simulink model "app_Main10msMgrrr"  (R2019b)
settings: Solver=FixedStepDiscrete  StartTime=0.0  StopTime=inf  FixedStep=0.01  RelTol=1e-3  EnableMultiTasking=on
PreLoadFcn:
  | try
  |    tapas_types('load');
  | catch
  |   disp('TAPAS WARNING: Tapas Types could not be loaded ...');
  | end
  | 
  | try
  |   app_types('load');
  | catch
  |   currdir =pwd;
  |   try
  |     cd('..\app_types\');
  |     app_types('load');
  |     cd(currdir);
  |   catch
  |     try
  |        cd('..\..\app_types\');
  |        app_types('load');
  |        cd(currdir);
  |     catch
  |        cd(currdir);
  |        disp('TAPAS WARNING: Application Types could not be loaded ...');
  |     end
  |   end
  |   try
  |       clear currdir;
  |   catch
  |      %Do nothing
  |   end
  | end
libraries: Lib_Rev2_Dvcu_IO x44, Lib_Rev2_Dvcu_Anlg x23, simulink x3, hdlsllib x1
settings Model: Creator=kmansour  LastModifiedBy=User
settings DataIOCC: LimitDataPoints=on  SaveFormat=Array  ReturnWorkspaceOutputs=off
settings OptimizationCC: LifeSpan=1  EfficientTunableParamExpr=on
settings DebuggingCC: AllowSymbolicDim=off  SFUnexpectedBacktrackingDiag=warning  SFNoUnconditionalDefaultTransitionDiag=warning  SFExecutionAtInitializationDiag=none  ArithmeticOperatorsInVariantConditions=warning
settings HardwareCC: ProdBitPerPointer=32  ProdBitPerSizeT=32  ProdBitPerPtrDiffT=32  ProdLargestAtomicInteger=Long  ProdLargestAtomicFloat=Double  ProdEndianess=BigEndian  ProdWordSize=32  ProdHWDeviceType=Texas Instruments->TMS570 Cortex-R4
settings ModelReferenceCC: ModelReferenceNumInstancesAllowed=Single  PropagateSignalLabelsOutOfModel=off
settings SFSimCC: SimUseLocalCustomCode=off  MATLABDynamicMemAlloc=off  CustomCodeUndefinedFunction=UseInterfaceOnly
settings RTWCC: SystemTargetFile=ert.tlc  GenCodeOnly=on  TemplateMakefile=ert_default_tmf  GenerateReport=on  RTWUseLocalCustomCode=off  IncludeHyperlinkInReport=on  LaunchReport=on  GenerateTraceInfo=on  GenerateTraceReport=on  GenerateTraceReportSl=on  GenerateTraceReportSf=on  GenerateTraceReportEml=on  CheckMdlBeforeBuild=Warning
settings CodeAppCC: IgnoreCustomStorageClasses=off  MaxIdLength=63  StateflowObjectComments=on
settings ERTTargetCC: MultiwordLength=2048  GenerateSampleERTMain=on  SuppressErrorStatus=on  GenerateASAP2=on  RTWCAPISignals=on  RTWCAPIParams=on  RTWCAPIStates=on  RTWCAPIRootIO=on  ERTSrcFileBannerTemplate=deMCD_code_template.cgt  ERTHdrFileBannerTemplate=deMCD_code_template.cgt  ERTDataSrcFileTemplate=deMCD_code_template.cgt  ERTDataHdrFileTemplate=deMCD_code_template.cgt  ERTCustomFileTemplate=example_file_process.tlc  ConvertIfToSwitch=off  SuppressUnreachableDefaultCases=off
settings ConfigComp: CovMetricSettings=dw  CovHtmlReporting=on  CovSaveCumulativeToWorkspaceVar=on  CovSaveSingleToWorkspaceVar=on  CovExternalEMLEnable=off

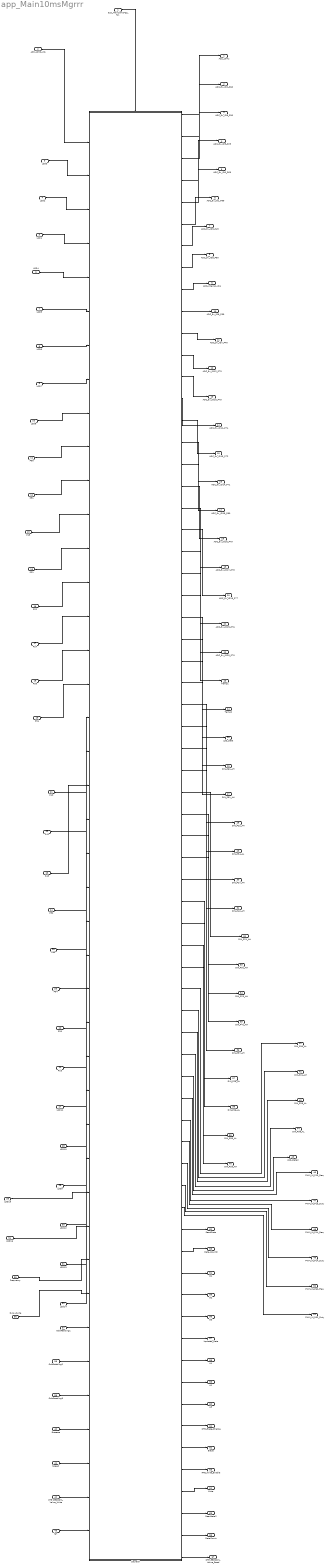
== system app_Main10msMgrrr ==
  app_Main10msMgr_fcn : Inport  SampleTime=10e-3  OutputFunctionCall=on
  APP_10MS_IN1 : Inport  Port=2
  LSD3 : Inport  Port=3
  LSD2 : Inport  Port=4
  LSD1 : Inport  Port=5
  LSD4 : Inport  Port=6
  LSD5 : Inport  Port=7
  LSD6 : Inport  Port=8
  LSD7 : Inport  Port=9
  LSD8 : Inport  Port=10
  P90 : Inport  Port=11
  P91 : Inport  Port=12
  P15 : Inport  Port=13
  P16 : Inport  Port=14
  P21 : Inport  Port=15
  P22 : Inport  Port=16
  P24 : Inport  Port=17
  P33 : Inport  Port=18
  P34 : Inport  Port=19
  P20 : Inport  Port=20
  P40 : Inport  Port=21
  P42 : Inport  Port=22
  P43 : Inport  Port=23
  P92 : Inport  Port=24
  P93 : Inport  Port=25
  P94 : Inport  Port=26
  LSD11 : Inport  Port=27
  LSD10 : Inport  Port=28
  LSD9 : Inport  Port=29
  LSD12 : Inport  Port=30
  LSD13 : Inport  Port=31
  LSD14 : Inport  Port=32
  LSD15 : Inport  Port=33
  LSD16 : Inport  Port=34
  Frequency : Inport  Port=35
  Duty_Cycle : Inport  Port=36
  OdoReading1 : Inport  Port=37
  OdoReading2 : Inport  Port=38
  OdoReading3 : Inport  Port=39
  Eraseee : Inport  Port=40
  Speed : Inport  Port=41
  RTE_EEPROM_Value_Write : Inport  Port=42
  Ign : Inport  Port=43
  Saurabh : Subsystem
      mask Display: image(('Devise Logo.JPG'),'center');
  App_10ms : Outport
  ADC_5v_ID2_P60 : Outport  Port=2
  ADC_5v_ID8_P30 : Outport  Port=3
  ADC_5v_ID9_P29 : Outport  Port=4
  ADC_5v_ID0_P69 : Outport  Port=5
  ADC_5v_ID1_P59 : Outport  Port=6
  ADC_5v_ID3_P49 : Outport  Port=7
  ADC_5v_ID5_P50 : Outport  Port=8
  ADC_Internal_ID4 : Outport  Port=9
  ADC_5v_ID6_P39 : Outport  Port=10
  ADC_5v_ID7_P40 : Outport  Port=11
  ADC_5v_ID12_P73 : Outport  Port=12
  ADC_5v_ID10_P75 : Outport  Port=13
  ADC_5v_ID11_P74 : Outport  Port=14
  ADC_5v_ID13_P72 : Outport  Port=15
  ADC_5v_ID14_P71 : Outport  Port=16
  ADC_5v_ID15_P80 : Outport  Port=17
  ADC_5v_ID16_P79 : Outport  Port=18
  ADC_5v_ID17_P78 : Outport  Port=19
  ADC_5v_ID18_P77 : Outport  Port=20
  ADC_5v_ID19_P76 : Outport  Port=21
  ADC_5v_ID20_P70 : Outport  Port=22
  Temp1 : Outport  Port=23
  Temp2 : Outport  Port=24
  LSD_Data : Outport  Port=25
  DIN_P61_AH : Outport  Port=26
  DIN_P51_AH : Outport  Port=27
  DIN_P22_AH : Outport  Port=28
  DIN_P34_AL : Outport  Port=29
  DIN_P27_AH : Outport  Port=30
  DIN_P42_AH : Outport  Port=31
  DIN_P21_AH : Outport  Port=32
  DIN_P31_AH : Outport  Port=33
  DIN_P23_AH : Outport  Port=34
  DIN_P41_AH : Outport  Port=35
  DIN_P37_AH : Outport  Port=36
  DIN_P25_AL : Outport  Port=37
  DIN_P26_AL : Outport  Port=38
  DIN_P35_AL : Outport  Port=39
  DIN_P33_AH : Outport  Port=40
  DIN_P36_AL : Outport  Port=41
  DIN_P24_AH : Outport  Port=42
  DIN_P28_AL : Outport  Port=43
  DIN_P38_AL : Outport  Port=44
  LSD_Data2 : Outport  Port=45
  PWM_IN_P13_Freq : Outport  Port=46
  PWM_IN_P13_Duty : Outport  Port=47
  PWM_IN_P14_Freq : Outport  Port=48
  PWM_IN_P14_Duty : Outport  Port=49
  PWM_IN_P62_Freq : Outport  Port=50
  PWM_IN_P62_Duty : Outport  Port=51
  ReadData : Outport  Port=52
  Data_Count2 : Outport  Port=53
  D1 : Outport  Port=54
  D2 : Outport  Port=55
  D3 : Outport  Port=56
  Updated_Data : Outport  Port=57
  A1 : Outport  Port=58
  A2 : Outport  Port=59
  A3 : Outport  Port=60
  RTE_Erase_Enable : Outport  Port=61
  Erase : Outport  Port=62
  RTE_Write_Enable : Outport  Port=63
  Write : Outport  Port=64
  Readdata2 : Outport  Port=65
  DataCount : Outport  Port=66
  RTE_EEPROM_Value_Read : Outport  Port=67
  wires:
  app_Main10msMgr_fcn/1 -> Saurabh/Trigger
  APP_10MS_IN1/1 -> Saurabh/1(APP_10MS_IN1)
  Saurabh/1(APP_10MS_OUT1) -> App_10ms/1
  Saurabh/5(ADC_5v_ID0_P69) -> ADC_5v_ID0_P69/1
  Saurabh/3(ADC_5v_ID8_P30) -> ADC_5v_ID8_P30/1
  Saurabh/4(ADC_5v_ID9_P29) -> ADC_5v_ID9_P29/1
  Saurabh/8(ADC_5v_ID5_P50) -> ADC_5v_ID5_P50/1
  Saurabh/7(ADC_5v_ID3_P49) -> ADC_5v_ID3_P49/1
  Saurabh/11(ADC_5v_ID7_P40) -> ADC_5v_ID7_P40/1
  Saurabh/2(ADC_5v_ID2_P60) -> ADC_5v_ID2_P60/1
  Saurabh/9(Power_Supply24v) -> ADC_Internal_ID4/1
  Saurabh/13(ADC_5v_ID10_P75) -> ADC_5v_ID10_P75/1
  Saurabh/6(ADC_5v_ID1_P59) -> ADC_5v_ID1_P59/1
  Saurabh/10(ADC_5v_ID6_P39) -> ADC_5v_ID6_P39/1
  Saurabh/12(ADC_5v_ID12_P73) -> ADC_5v_ID12_P73/1
  Saurabh/19(ADC_5v_ID17_P78) -> ADC_5v_ID17_P78/1
  Saurabh/17(ADC_5v_ID15_P80) -> ADC_5v_ID15_P80/1
  Saurabh/20(ADC_5v_ID18_P77) -> ADC_5v_ID18_P77/1
  Saurabh/21(ADC_5v_ID19_P76) -> ADC_5v_ID19_P76/1
  Saurabh/22(ADC_5v_ID20_P70) -> ADC_5v_ID20_P70/1
  Saurabh/16(ADC_5v_ID14_P71) -> ADC_5v_ID14_P71/1
  Saurabh/14(ADC_5v_ID11_P74) -> ADC_5v_ID11_P74/1
  Saurabh/18(ADC_5v_ID16_P79) -> ADC_5v_ID16_P79/1
  Saurabh/15(ADC_5v_ID13_P72) -> ADC_5v_ID13_P72/1
  Saurabh/23(Temp1) -> Temp1/1
  Saurabh/24(Temp2) -> Temp2/1
  LSD1/1 -> Saurabh/4(LSD1)
  LSD2/1 -> Saurabh/3(LSD2)
  LSD3/1 -> Saurabh/2(LSD3)
  LSD4/1 -> Saurabh/5(LSD4)
  LSD8/1 -> Saurabh/9(LSD8)
  LSD5/1 -> Saurabh/6(LSD5)
  LSD7/1 -> Saurabh/8(LSD7)
  LSD6/1 -> Saurabh/7(LSD6)
  Saurabh/25(LSD_Data) -> LSD_Data/1
  P90/1 -> Saurabh/10(P90)
  P91/1 -> Saurabh/11(P91)
  P15/1 -> Saurabh/12(P15)
  P16/1 -> Saurabh/25(P16)
  P21/1 -> Saurabh/13(P21)
  P22/1 -> Saurabh/14(P22)
  P24/1 -> Saurabh/15(P24)
  P33/1 -> Saurabh/16(P33)
  P34/1 -> Saurabh/17(P34)
  P20/1 -> Saurabh/24(P20)
  P93/1 -> Saurabh/22(P93)
  P42/1 -> Saurabh/19(P42)
  P43/1 -> Saurabh/20(P43)
  P40/1 -> Saurabh/18(P40)
  P92/1 -> Saurabh/21(P92)
  P94/1 -> Saurabh/23(P94)
  Saurabh/34(DIN_P23_AH) -> DIN_P23_AH/1
  Saurabh/29(DIN_P34_AL) -> DIN_P34_AL/1
  Saurabh/28(DIN_P22_AH) -> DIN_P22_AH/1
  Saurabh/31(DIN_P42_AH) -> DIN_P42_AH/1
  Saurabh/27(DIN_P51_AH) -> DIN_P51_AH/1
  Saurabh/33(DIN_P31_AH) -> DIN_P31_AH/1
  Saurabh/35(DIN_P41_AH) -> DIN_P41_AH/1
  Saurabh/32(DIN_P21_AH) -> DIN_P21_AH/1
  Saurabh/26(DIN_P61_AH) -> DIN_P61_AH/1
  Saurabh/30(DIN_P27_AH) -> DIN_P27_AH/1
  Saurabh/44(DIN_P38_AL) -> DIN_P38_AL/1
  Saurabh/36(DIN_P37_AH) -> DIN_P37_AH/1
  Saurabh/42(DIN_P24_AH) -> DIN_P24_AH/1
  Saurabh/38(DIN_P26_AL) -> DIN_P26_AL/1
  Saurabh/39(DIN_P35_AL) -> DIN_P35_AL/1
  Saurabh/43(DIN_P28_AL) -> DIN_P28_AL/1
  Saurabh/40(DIN_P33_AH) -> DIN_P33_AH/1
  Saurabh/37(DIN_P25_AL) -> DIN_P25_AL/1
  Saurabh/41(DIN_P36_AL) -> DIN_P36_AL/1
  LSD11/1 -> Saurabh/26(LSD11)
  LSD10/1 -> Saurabh/27(LSD10)
  LSD9/1 -> Saurabh/28(LSD9)
  LSD12/1 -> Saurabh/29(LSD12)
  LSD15/1 -> Saurabh/32(LSD15)
  LSD13/1 -> Saurabh/30(LSD13)
  LSD16/1 -> Saurabh/33(LSD16)
  LSD14/1 -> Saurabh/31(LSD14)
  Saurabh/45(LSD_Data2) -> LSD_Data2/1
  Saurabh/46(PWM_IN_P13_Freq) -> PWM_IN_P13_Freq/1
  Saurabh/47(PWM_IN_P13_Duty) -> PWM_IN_P13_Duty/1
  Duty_Cycle/1 -> Saurabh/35(Duty_Cycle)
  Frequency/1 -> Saurabh/34(Frequency)
  Saurabh/51(PWM_IN_P62_Duty) -> PWM_IN_P62_Duty/1
  Saurabh/50(PWM_IN_P62_Freq) -> PWM_IN_P62_Freq/1
  Saurabh/49(PWM_IN_P14_Duty) -> PWM_IN_P14_Duty/1
  Saurabh/48(PWM_IN_P14_Freq) -> PWM_IN_P14_Freq/1
  OdoReading1/1 -> Saurabh/36(OdoReading1)
  RTE_EEPROM_Value_Write/1 -> Saurabh/41(RTE_EEPROM_Value_Write)
  Speed/1 -> Saurabh/40(Speed)
  Eraseee/1 -> Saurabh/39(Eraseee)
  Ign/1 -> Saurabh/42(Ign)
  OdoReading3/1 -> Saurabh/38(OdoReading3)
  OdoReading2/1 -> Saurabh/37(OdoReading2)
  Saurabh/52(ReadData) -> ReadData/1
  Saurabh/53(Data_Count2) -> Data_Count2/1
  Saurabh/56(D3) -> D3/1
  Saurabh/54(D1) -> D1/1
  Saurabh/55(D2) -> D2/1
  Saurabh/58(A1) -> A1/1
  Saurabh/59(A2) -> A2/1
  Saurabh/60(A3) -> A3/1
  Saurabh/57(Updated_Data) -> Updated_Data/1
  Saurabh/61(RTE_Erase_Enable) -> RTE_Erase_Enable/1
  Saurabh/62(Erase) -> Erase/1
  Saurabh/63(RTE_Write_Enable) -> RTE_Write_Enable/1
  Saurabh/64(Write) -> Write/1
  Saurabh/65(Readdata2) -> Readdata2/1
  Saurabh/66(DataCount) -> DataCount/1
  Saurabh/67(RTE_EEPROM_Value_Read) -> RTE_EEPROM_Value_Read/1

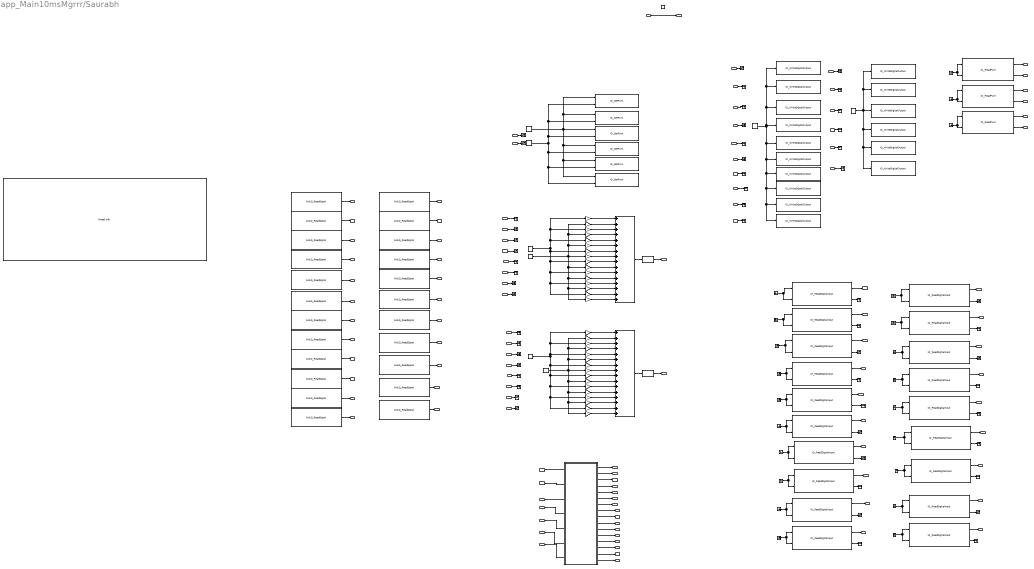
== system app_Main10msMgrrr/Saurabh ==
  note: EPROM
  note: Inputs
  note: HSD
  note: PWM
  note: ADC
  note: (C) 2020-2021 Devise Electronics Pvt Ltd
      | All rights reserved.
      |
      | All data and information contained in or disclosed by this document is confidential and proprietary information of Devise Electronics Pvt Ltd and all rights therein are expressly reserved. By accepting this material the recipient agrees that this material and the information contained therein is held in confidence and in trust and will not be used, copied, reproduced in whole or in part, nor its contents revealed in any manner to others without the express written permission of Devise Electronics Pvt Ltd
      |
      | Author: Vinay Pawar | Devise E-106
      |
      | Devise Electronics Pvt Ltd
      | Pune,
      | India
      | E-mail: Shekhar.malani@deviseelectronics.com
  note: LSD1
  note: LSD2
  APP_10MS_IN1 : Inport
  LSD3 : Inport  Port=2
  LSD2 : Inport  Port=3
  LSD1 : Inport  Port=4
  LSD4 : Inport  Port=5
  LSD5 : Inport  Port=6
  LSD6 : Inport  Port=7
  LSD7 : Inport  Port=8
  LSD8 : Inport  Port=9
  P90 : Inport  Port=10
  P91 : Inport  Port=11
  P15 : Inport  Port=12
  P21 : Inport  Port=13
  P22 : Inport  Port=14
  P24 : Inport  Port=15
  P33 : Inport  Port=16
  P34 : Inport  Port=17
  P40 : Inport  Port=18
  P42 : Inport  Port=19
  P43 : Inport  Port=20
  P92 : Inport  Port=21
  P93 : Inport  Port=22
  P94 : Inport  Port=23
  P20 : Inport  Port=24
  P16 : Inport  Port=25
  LSD11 : Inport  Port=26
  LSD10 : Inport  Port=27
  LSD9 : Inport  Port=28
  LSD12 : Inport  Port=29
  LSD13 : Inport  Port=30
  LSD14 : Inport  Port=31
  LSD15 : Inport  Port=32
  LSD16 : Inport  Port=33
  Frequency : Inport  Port=34
  Duty_Cycle : Inport  Port=35
  OdoReading1 : Inport  Port=36
  OdoReading2 : Inport  Port=37
  OdoReading3 : Inport  Port=38
  Eraseee : Inport  Port=39
  Speed : Inport  Port=40
  RTE_EEPROM_Value_Write : Inport  Port=41
  Ign : Inport  Port=42
  Trigger : TriggerPort  TriggerType=function-call  VariantControl=Variant  SampleTimeType=periodic  SampleTime=-1  PortDimensions=1
  ANLG_ReadSignal : Lib_Rev2_Dvcu_Anlg/ANLG_ReadSignal  PARAM_ID=ECU_ANLG_ADC_5V_P60
      settings: SourceProductName=deMCD - Rev2_Dvcu
  ANLG_ReadSignal1 : Lib_Rev2_Dvcu_Anlg/ANLG_ReadSignal  PARAM_ID=ECU_ANLG_ADC_5V_P30
      settings: SourceProductName=deMCD - Rev2_Dvcu
  ANLG_ReadSignal10 : Lib_Rev2_Dvcu_Anlg/ANLG_ReadSignal  PARAM_ID=ECU_ANLG_ADC_5V_P73
      settings: SourceProductName=deMCD - Rev2_Dvcu
  ANLG_ReadSignal11 : Lib_Rev2_Dvcu_Anlg/ANLG_ReadSignal  PARAM_ID=ECU_ANLG_ADC_5V_P75
      settings: SourceProductName=deMCD - Rev2_Dvcu
  ANLG_ReadSignal12 : Lib_Rev2_Dvcu_Anlg/ANLG_ReadSignal  PARAM_ID=ECU_ANLG_ADC_5V_P74
      settings: SourceProductName=deMCD - Rev2_Dvcu
  ANLG_ReadSignal13 : Lib_Rev2_Dvcu_Anlg/ANLG_ReadSignal  PARAM_ID=ECU_ANLG_ADC_5V_P72
      settings: SourceProductName=deMCD - Rev2_Dvcu
  ANLG_ReadSignal14 : Lib_Rev2_Dvcu_Anlg/ANLG_ReadSignal  PARAM_ID=ECU_ANLG_ADC_5V_P71
      settings: SourceProductName=deMCD - Rev2_Dvcu
  ANLG_ReadSignal15 : Lib_Rev2_Dvcu_Anlg/ANLG_ReadSignal  PARAM_ID=ECU_ANLG_ADC_5V_P80
      settings: SourceProductName=deMCD - Rev2_Dvcu
  ANLG_ReadSignal16 : Lib_Rev2_Dvcu_Anlg/ANLG_ReadSignal  PARAM_ID=ECU_ANLG_ADC_5V_P79
      settings: SourceProductName=deMCD - Rev2_Dvcu
  ANLG_ReadSignal17 : Lib_Rev2_Dvcu_Anlg/ANLG_ReadSignal  PARAM_ID=ECU_ANLG_ADC_5V_P78
      settings: SourceProductName=deMCD - Rev2_Dvcu
  ANLG_ReadSignal18 : Lib_Rev2_Dvcu_Anlg/ANLG_ReadSignal  PARAM_ID=ECU_ANLG_ADC_5V_P77
      settings: SourceProductName=deMCD - Rev2_Dvcu
  ANLG_ReadSignal19 : Lib_Rev2_Dvcu_Anlg/ANLG_ReadSignal  PARAM_ID=ECU_ANLG_ADC_5V_P76
      settings: SourceProductName=deMCD - Rev2_Dvcu
  ANLG_ReadSignal2 : Lib_Rev2_Dvcu_Anlg/ANLG_ReadSignal  PARAM_ID=ECU_ANLG_ADC_5V_P29
      settings: SourceProductName=deMCD - Rev2_Dvcu
  ANLG_ReadSignal20 : Lib_Rev2_Dvcu_Anlg/ANLG_ReadSignal  PARAM_ID=ECU_ANLG_ADC_5V_P70
      settings: SourceProductName=deMCD - Rev2_Dvcu
  ANLG_ReadSignal22 : Lib_Rev2_Dvcu_Anlg/ANLG_ReadSignal  PARAM_ID=ECU_ANLG_TEMP_SENSOR1
      settings: SourceProductName=deMCD - Rev2_Dvcu
  ANLG_ReadSignal23 : Lib_Rev2_Dvcu_Anlg/ANLG_ReadSignal  PARAM_ID=ECU_ANLG_TEMP_SENSOR2
      settings: SourceProductName=deMCD - Rev2_Dvcu
  ANLG_ReadSignal3 : Lib_Rev2_Dvcu_Anlg/ANLG_ReadSignal  PARAM_ID=ECU_ANLG_ADC_5V_P69
      settings: SourceProductName=deMCD - Rev2_Dvcu
  ANLG_ReadSignal4 : Lib_Rev2_Dvcu_Anlg/ANLG_ReadSignal  PARAM_ID=ECU_ANLG_ADC_5V_P59
      settings: SourceProductName=deMCD - Rev2_Dvcu
  ANLG_ReadSignal5 : Lib_Rev2_Dvcu_Anlg/ANLG_ReadSignal  PARAM_ID=ECU_ANLG_ADC_5V_P49
      settings: SourceProductName=deMCD - Rev2_Dvcu
  ANLG_ReadSignal6 : Lib_Rev2_Dvcu_Anlg/ANLG_ReadSignal  PARAM_ID=ECU_ANLG_ADC_5V_P50
      settings: SourceProductName=deMCD - Rev2_Dvcu
  ANLG_ReadSignal7 : Lib_Rev2_Dvcu_Anlg/ANLG_ReadSignal  PARAM_ID=ECU_ANLG_POWER_SUPPLY24V
      settings: SourceProductName=deMCD - Rev2_Dvcu
  ANLG_ReadSignal8 : Lib_Rev2_Dvcu_Anlg/ANLG_ReadSignal  PARAM_ID=ECU_ANLG_ADC_5V_P39
      settings: SourceProductName=deMCD - Rev2_Dvcu
  ANLG_ReadSignal9 : Lib_Rev2_Dvcu_Anlg/ANLG_ReadSignal  PARAM_ID=ECU_ANLG_ADC_5V_P40
      settings: SourceProductName=deMCD - Rev2_Dvcu
  Add1 : Sum  Inputs=++++++++++++++++
  Add2 : Sum  Inputs=++++++++++++++++
  Constant : Constant  Value=1000
  Constant1 : Constant  Value=0
  Constant17 : Constant  Value=0
  Constant{2..5} (4 alike) : Constant
  Constant6 : Constant  Value=100
  Data Type Conversion1 : DataTypeConversion  OutDataTypeStr=uint16
  Data Type Conversion2 : DataTypeConversion  OutDataTypeStr=uint16
  Gain : Gain
  Gain1 : Gain  Gain=2
  Gain10 : Gain  Gain=1024
  Gain11 : Gain  Gain=2048
  Gain12 : Gain  Gain=4096
  Gain13 : Gain  Gain=8192
  Gain14 : Gain  Gain=16384
  Gain15 : Gain  Gain=32768
  Gain16 : Gain
  Gain17 : Gain  Gain=2
  Gain18 : Gain  Gain=1024
  Gain19 : Gain  Gain=2048
  Gain2 : Gain  Gain=4
  Gain20 : Gain  Gain=4096
  Gain21 : Gain  Gain=8192
  Gain22 : Gain  Gain=16384
  Gain23 : Gain  Gain=32768
  Gain24 : Gain  Gain=4
  Gain25 : Gain  Gain=8
  Gain26 : Gain  Gain=16
  Gain27 : Gain  Gain=32
  Gain28 : Gain  Gain=64
  Gain29 : Gain  Gain=128
  Gain3 : Gain  Gain=8
  Gain30 : Gain  Gain=256
  Gain31 : Gain  Gain=512
  Gain4 : Gain  Gain=16
  Gain5 : Gain  Gain=32
  Gain6 : Gain  Gain=64
  Gain7 : Gain  Gain=128
  Gain8 : Gain  Gain=256
  Gain9 : Gain  Gain=512
  Ground{,1..21} (22 alike) : Ground
  IO_ReadDigitalInput : Lib_Rev2_Dvcu_IO/IO_ReadDigitalInput  PARAM_ID=ECU_DIN_AUX_61_H_DI
      settings: SourceProductName=deMCD - Rev2_Dvcu
  IO_ReadDigitalInput1 : Lib_Rev2_Dvcu_IO/IO_ReadDigitalInput  PARAM_ID=ECU_DIN_AUX_51_H_DI
      settings: SourceProductName=deMCD - Rev2_Dvcu
  IO_ReadDigitalInput10 : Lib_Rev2_Dvcu_IO/IO_ReadDigitalInput  PARAM_ID=ECU_DIN_AUX_26_L_DI
      settings: SourceProductName=deMCD - Rev2_Dvcu
  IO_ReadDigitalInput11 : Lib_Rev2_Dvcu_IO/IO_ReadDigitalInput  PARAM_ID=ECU_DIN_AUX_35_L_DI
      settings: SourceProductName=deMCD - Rev2_Dvcu
  IO_ReadDigitalInput12 : Lib_Rev2_Dvcu_IO/IO_ReadDigitalInput  PARAM_ID=ECU_DIN_AUX_33_H_DI
      settings: SourceProductName=deMCD - Rev2_Dvcu
  IO_ReadDigitalInput13 : Lib_Rev2_Dvcu_IO/IO_ReadDigitalInput  PARAM_ID=ECU_DIN_AUX_36_L_DI
      settings: SourceProductName=deMCD - Rev2_Dvcu
  IO_ReadDigitalInput14 : Lib_Rev2_Dvcu_IO/IO_ReadDigitalInput  PARAM_ID=ECU_DIN_AUX_24_H_DI
      settings: SourceProductName=deMCD - Rev2_Dvcu
  IO_ReadDigitalInput15 : Lib_Rev2_Dvcu_IO/IO_ReadDigitalInput  PARAM_ID=ECU_DIN_AUX_23_H_DI
      settings: SourceProductName=deMCD - Rev2_Dvcu
  IO_ReadDigitalInput16 : Lib_Rev2_Dvcu_IO/IO_ReadDigitalInput  PARAM_ID=ECU_DIN_AUX_28_L_DI
      settings: SourceProductName=deMCD - Rev2_Dvcu
  IO_ReadDigitalInput17 : Lib_Rev2_Dvcu_IO/IO_ReadDigitalInput  PARAM_ID=ECU_DIN_AUX_41_H_DI
      settings: SourceProductName=deMCD - Rev2_Dvcu
  IO_ReadDigitalInput18 : Lib_Rev2_Dvcu_IO/IO_ReadDigitalInput  PARAM_ID=ECU_DIN_AUX_38_L_DI
      settings: SourceProductName=deMCD - Rev2_Dvcu
  IO_ReadDigitalInput2 : Lib_Rev2_Dvcu_IO/IO_ReadDigitalInput  PARAM_ID=ECU_DIN_AUX_22_H_DI
      settings: SourceProductName=deMCD - Rev2_Dvcu
  IO_ReadDigitalInput3 : Lib_Rev2_Dvcu_IO/IO_ReadDigitalInput  PARAM_ID=ECU_DIN_AUX_34_L_DI
      settings: SourceProductName=deMCD - Rev2_Dvcu
  IO_ReadDigitalInput4 : Lib_Rev2_Dvcu_IO/IO_ReadDigitalInput  PARAM_ID=ECU_DIN_AUX_27_H_DI
      settings: SourceProductName=deMCD - Rev2_Dvcu
  IO_ReadDigitalInput5 : Lib_Rev2_Dvcu_IO/IO_ReadDigitalInput  PARAM_ID=ECU_DIN_AUX_42_H_DI
      settings: SourceProductName=deMCD - Rev2_Dvcu
  IO_ReadDigitalInput6 : Lib_Rev2_Dvcu_IO/IO_ReadDigitalInput  PARAM_ID=ECU_DIN_AUX_21_H_DI
      settings: SourceProductName=deMCD - Rev2_Dvcu
  IO_ReadDigitalInput7 : Lib_Rev2_Dvcu_IO/IO_ReadDigitalInput  PARAM_ID=ECU_DIN_AUX_31_H_DI
      settings: SourceProductName=deMCD - Rev2_Dvcu
  IO_ReadDigitalInput8 : Lib_Rev2_Dvcu_IO/IO_ReadDigitalInput  PARAM_ID=ECU_DIN_AUX_37_H_DI
      settings: SourceProductName=deMCD - Rev2_Dvcu
  IO_ReadDigitalInput9 : Lib_Rev2_Dvcu_IO/IO_ReadDigitalInput  PARAM_ID=ECU_DIN_AUX_25_L_DI
      settings: SourceProductName=deMCD - Rev2_Dvcu
  IO_ReadPwm : Lib_Rev2_Dvcu_IO/IO_ReadPwm  PARAM_ID=ECU_PIN_NONAME_PIN_P13
      settings: SourceProductName=deMCD - Rev2_Dvcu
  IO_ReadPwm1 : Lib_Rev2_Dvcu_IO/IO_ReadPwm  PARAM_ID=ECU_PIN_NONAME_PIN_P14
      settings: SourceProductName=deMCD - Rev2_Dvcu
  IO_ReadPwm2 : Lib_Rev2_Dvcu_IO/IO_ReadPwm  PARAM_ID=ECU_PIN_NONAME_PIN_P62
      settings: SourceProductName=deMCD - Rev2_Dvcu
  IO_SetPwm : Lib_Rev2_Dvcu_IO/IO_SetPwm  PARAM_ID=ECU_POUT_PWM_POUT_ID_0
      settings: SourceProductName=deMCD - Rev2_Dvcu
  IO_SetPwm1 : Lib_Rev2_Dvcu_IO/IO_SetPwm  PARAM_ID=ECU_POUT_PWM_POUT_ID_1
      settings: SourceProductName=deMCD - Rev2_Dvcu
  IO_SetPwm2 : Lib_Rev2_Dvcu_IO/IO_SetPwm  PARAM_ID=ECU_POUT_PWM_POUT_ID_2
      settings: SourceProductName=deMCD - Rev2_Dvcu
  IO_SetPwm3 : Lib_Rev2_Dvcu_IO/IO_SetPwm  PARAM_ID=ECU_POUT_PWM_POUT_ID_3
      settings: SourceProductName=deMCD - Rev2_Dvcu
  IO_SetPwm4 : Lib_Rev2_Dvcu_IO/IO_SetPwm  PARAM_ID=ECU_POUT_PWM_POUT_ID_4
      settings: SourceProductName=deMCD - Rev2_Dvcu
  IO_SetPwm5 : Lib_Rev2_Dvcu_IO/IO_SetPwm  PARAM_ID=ECU_POUT_PWM_POUT_ID_5
      settings: SourceProductName=deMCD - Rev2_Dvcu
  IO_WriteDigitalOutput : Lib_Rev2_Dvcu_IO/IO_WriteDigitalOutput  PARAM_ID=ECU_DOUT_NONAME_PIN_P90
      settings: SourceProductName=deMCD - Rev2_Dvcu
  IO_WriteDigitalOutput1 : Lib_Rev2_Dvcu_IO/IO_WriteDigitalOutput  PARAM_ID=ECU_DOUT_NONAME_PIN_P91
      settings: SourceProductName=deMCD - Rev2_Dvcu
  IO_WriteDigitalOutput10 : Lib_Rev2_Dvcu_IO/IO_WriteDigitalOutput  PARAM_ID=ECU_DOUT_NONAME_PIN_P40
      settings: SourceProductName=deMCD - Rev2_Dvcu
  IO_WriteDigitalOutput11 : Lib_Rev2_Dvcu_IO/IO_WriteDigitalOutput  PARAM_ID=ECU_DOUT_NONAME_PIN_P42
      settings: SourceProductName=deMCD - Rev2_Dvcu
  IO_WriteDigitalOutput12 : Lib_Rev2_Dvcu_IO/IO_WriteDigitalOutput  PARAM_ID=ECU_DOUT_NONAME_PIN_P43
      settings: SourceProductName=deMCD - Rev2_Dvcu
  IO_WriteDigitalOutput13 : Lib_Rev2_Dvcu_IO/IO_WriteDigitalOutput  PARAM_ID=ECU_DOUT_NONAME_PIN_P92
      settings: SourceProductName=deMCD - Rev2_Dvcu
  IO_WriteDigitalOutput14 : Lib_Rev2_Dvcu_IO/IO_WriteDigitalOutput  PARAM_ID=ECU_DOUT_NONAME_PIN_P93
      settings: SourceProductName=deMCD - Rev2_Dvcu
  IO_WriteDigitalOutput15 : Lib_Rev2_Dvcu_IO/IO_WriteDigitalOutput  PARAM_ID=ECU_DOUT_NONAME_PIN_P94
      settings: SourceProductName=deMCD - Rev2_Dvcu
  IO_WriteDigitalOutput2 : Lib_Rev2_Dvcu_IO/IO_WriteDigitalOutput  PARAM_ID=ECU_DOUT_NONAME_PIN_P15
      settings: SourceProductName=deMCD - Rev2_Dvcu
  IO_WriteDigitalOutput3 : Lib_Rev2_Dvcu_IO/IO_WriteDigitalOutput  PARAM_ID=ECU_DOUT_NONAME_PIN_P16
      settings: SourceProductName=deMCD - Rev2_Dvcu
  IO_WriteDigitalOutput4 : Lib_Rev2_Dvcu_IO/IO_WriteDigitalOutput  PARAM_ID=ECU_DOUT_NONAME_PIN_P20
      settings: SourceProductName=deMCD - Rev2_Dvcu
  IO_WriteDigitalOutput5 : Lib_Rev2_Dvcu_IO/IO_WriteDigitalOutput  PARAM_ID=ECU_DOUT_NONAME_PIN_P21
      settings: SourceProductName=deMCD - Rev2_Dvcu
  IO_WriteDigitalOutput6 : Lib_Rev2_Dvcu_IO/IO_WriteDigitalOutput  PARAM_ID=ECU_DOUT_NONAME_PIN_P22
      settings: SourceProductName=deMCD - Rev2_Dvcu
  IO_WriteDigitalOutput7 : Lib_Rev2_Dvcu_IO/IO_WriteDigitalOutput  PARAM_ID=ECU_DOUT_NONAME_PIN_P24
      settings: SourceProductName=deMCD - Rev2_Dvcu
  IO_WriteDigitalOutput8 : Lib_Rev2_Dvcu_IO/IO_WriteDigitalOutput  PARAM_ID=ECU_DOUT_NONAME_PIN_P33
      settings: SourceProductName=deMCD - Rev2_Dvcu
  IO_WriteDigitalOutput9 : Lib_Rev2_Dvcu_IO/IO_WriteDigitalOutput  PARAM_ID=ECU_DOUT_NONAME_PIN_P34
      settings: SourceProductName=deMCD - Rev2_Dvcu
  Model Info : simulink/Model-Wide Utilities/Model Info  Frame=on  DisplayStringWithTags=|  HorizontalTextAlignment=Left  LeftAlignmentValue=0.02
      | File Name: app_Main10msMgr.slx
      |   Description: 
      |   Author: Saurabh kulkarni
      | 
      |   Modified date/ Time: %<ModifiedDate>
      |   Last Modified date/ Time: %<LastModificationDate>
  Subsystem1 : Subsystem
  Terminator{,1..52} (53 alike) : Terminator
  APP_10MS_OUT1 : Outport
  ADC_5v_ID2_P60 : Outport  Port=2
  ADC_5v_ID8_P30 : Outport  Port=3
  ADC_5v_ID9_P29 : Outport  Port=4
  ADC_5v_ID0_P69 : Outport  Port=5
  ADC_5v_ID1_P59 : Outport  Port=6
  ADC_5v_ID3_P49 : Outport  Port=7
  ADC_5v_ID5_P50 : Outport  Port=8
  Power_Supply24v : Outport  Port=9
  ADC_5v_ID6_P39 : Outport  Port=10
  ADC_5v_ID7_P40 : Outport  Port=11
  ADC_5v_ID12_P73 : Outport  Port=12
  ADC_5v_ID10_P75 : Outport  Port=13
  ADC_5v_ID11_P74 : Outport  Port=14
  ADC_5v_ID13_P72 : Outport  Port=15
  ADC_5v_ID14_P71 : Outport  Port=16
  ADC_5v_ID15_P80 : Outport  Port=17
  ADC_5v_ID16_P79 : Outport  Port=18
  ADC_5v_ID17_P78 : Outport  Port=19
  ADC_5v_ID18_P77 : Outport  Port=20
  ADC_5v_ID19_P76 : Outport  Port=21
  ADC_5v_ID20_P70 : Outport  Port=22
  Temp1 : Outport  Port=23
  Temp2 : Outport  Port=24
  LSD_Data : Outport  Port=25
  DIN_P61_AH : Outport  Port=26
  DIN_P51_AH : Outport  Port=27
  DIN_P22_AH : Outport  Port=28
  DIN_P34_AL : Outport  Port=29
  DIN_P27_AH : Outport  Port=30
  DIN_P42_AH : Outport  Port=31
  DIN_P21_AH : Outport  Port=32
  DIN_P31_AH : Outport  Port=33
  DIN_P23_AH : Outport  Port=34
  DIN_P41_AH : Outport  Port=35
  DIN_P37_AH : Outport  Port=36
  DIN_P25_AL : Outport  Port=37
  DIN_P26_AL : Outport  Port=38
  DIN_P35_AL : Outport  Port=39
  DIN_P33_AH : Outport  Port=40
  DIN_P36_AL : Outport  Port=41
  DIN_P24_AH : Outport  Port=42
  DIN_P28_AL : Outport  Port=43
  DIN_P38_AL : Outport  Port=44
  LSD_Data2 : Outport  Port=45
  PWM_IN_P13_Freq : Outport  Port=46
  PWM_IN_P13_Duty : Outport  Port=47
  PWM_IN_P14_Freq : Outport  Port=48
  PWM_IN_P14_Duty : Outport  Port=49
  PWM_IN_P62_Freq : Outport  Port=50
  PWM_IN_P62_Duty : Outport  Port=51
  ReadData : Outport  Port=52
  Data_Count2 : Outport  Port=53
  D1 : Outport  Port=54
  D2 : Outport  Port=55
  D3 : Outport  Port=56
  Updated_Data : Outport  Port=57
  A1 : Outport  Port=58
  A2 : Outport  Port=59
  A3 : Outport  Port=60
  RTE_Erase_Enable : Outport  Port=61
  Erase : Outport  Port=62
  RTE_Write_Enable : Outport  Port=63
  Write : Outport  Port=64
  Readdata2 : Outport  Port=65
  DataCount : Outport  Port=66
  RTE_EEPROM_Value_Read : Outport  Port=67
  wires:
  APP_10MS_IN1/1 -> APP_10MS_OUT1/1
  ? -> ?
  ANLG_ReadSignal/1 -> ADC_5v_ID2_P60/1
  ANLG_ReadSignal1/1 -> ADC_5v_ID8_P30/1
  ANLG_ReadSignal2/1 -> ADC_5v_ID9_P29/1
  ANLG_ReadSignal3/1 -> ADC_5v_ID0_P69/1
  ANLG_ReadSignal4/1 -> ADC_5v_ID1_P59/1
  ANLG_ReadSignal5/1 -> ADC_5v_ID3_P49/1
  ANLG_ReadSignal6/1 -> ADC_5v_ID5_P50/1
  ANLG_ReadSignal7/1 -> Power_Supply24v/1
  ANLG_ReadSignal8/1 -> ADC_5v_ID6_P39/1
  ANLG_ReadSignal9/1 -> ADC_5v_ID7_P40/1
  ANLG_ReadSignal10/1 -> ADC_5v_ID12_P73/1
  ANLG_ReadSignal11/1 -> ADC_5v_ID10_P75/1
  ANLG_ReadSignal12/1 -> ADC_5v_ID11_P74/1
  ANLG_ReadSignal13/1 -> ADC_5v_ID13_P72/1
  ANLG_ReadSignal14/1 -> ADC_5v_ID14_P71/1
  ANLG_ReadSignal15/1 -> ADC_5v_ID15_P80/1
  ANLG_ReadSignal16/1 -> ADC_5v_ID16_P79/1
  ANLG_ReadSignal17/1 -> ADC_5v_ID17_P78/1
  ANLG_ReadSignal18/1 -> ADC_5v_ID18_P77/1
  ANLG_ReadSignal19/1 -> ADC_5v_ID19_P76/1
  ANLG_ReadSignal20/1 -> ADC_5v_ID20_P70/1
  ANLG_ReadSignal22/1 -> Temp1/1
  ANLG_ReadSignal23/1 -> Temp2/1
  Constant/1 -> IO_SetPwm5/1, IO_SetPwm4/1, IO_SetPwm3/1, IO_SetPwm2/1, IO_SetPwm1/1, IO_SetPwm/1
  Constant6/1 -> IO_SetPwm3/2, IO_SetPwm5/2, IO_SetPwm4/2, IO_SetPwm/2, IO_SetPwm1/2, IO_SetPwm2/2
  Gain2/1 -> Add1/14
  Constant17/1 -> Gain4/1, Gain2/1, Gain/1, Gain6/1, Gain10/1, Gain12/1, Gain14/1, Gain8/1
  Gain15/1 -> Add1/1
  Gain14/1 -> Add1/2
  Gain5/1 -> Add1/11
  Gain4/1 -> Add1/12
  Gain/1 -> Add1/16
  Add1/1 -> Data Type Conversion1/1
  Gain6/1 -> Add1/10
  Data Type Conversion1/1 -> LSD_Data/1
  Gain1/1 -> Add1/15
  Gain13/1 -> Add1/3
  Gain9/1 -> Add1/7
  Gain8/1 -> Add1/8
  Gain7/1 -> Add1/9
  Gain3/1 -> Add1/13
  Gain11/1 -> Add1/5
  Gain10/1 -> Add1/6
  Gain12/1 -> Add1/4
  IO_ReadDigitalInput/1 -> DIN_P61_AH/1
  IO_ReadDigitalInput1/1 -> DIN_P51_AH/1
  IO_ReadDigitalInput2/1 -> DIN_P22_AH/1
  IO_ReadDigitalInput3/1 -> DIN_P34_AL/1
  IO_ReadDigitalInput4/1 -> DIN_P27_AH/1
  IO_ReadDigitalInput5/1 -> DIN_P42_AH/1
  IO_ReadDigitalInput6/1 -> DIN_P21_AH/1
  IO_ReadDigitalInput7/1 -> DIN_P31_AH/1
  IO_ReadDigitalInput17/1 -> DIN_P41_AH/1
  IO_ReadDigitalInput15/1 -> DIN_P23_AH/1
  IO_ReadDigitalInput9/1 -> DIN_P25_AL/1
  IO_ReadDigitalInput8/1 -> DIN_P37_AH/1
  IO_ReadDigitalInput11/1 -> DIN_P35_AL/1
  IO_ReadDigitalInput10/1 -> DIN_P26_AL/1
  IO_ReadDigitalInput13/1 -> DIN_P36_AL/1
  IO_ReadDigitalInput12/1 -> DIN_P33_AH/1
  IO_ReadDigitalInput16/1 -> DIN_P28_AL/1
  IO_ReadDigitalInput14/1 -> DIN_P24_AH/1
  IO_ReadDigitalInput18/1 -> DIN_P38_AL/1
  IO_ReadDigitalInput/2 -> Terminator/1
  Ground/1 -> IO_ReadDigitalInput/2, IO_ReadDigitalInput/1
  Ground1/1 -> IO_ReadDigitalInput1/2, IO_ReadDigitalInput1/1
  IO_ReadDigitalInput1/2 -> Terminator1/1
  Ground2/1 -> IO_ReadDigitalInput2/2, IO_ReadDigitalInput2/1
  Ground3/1 -> IO_ReadDigitalInput3/2, IO_ReadDigitalInput3/1
  Ground4/1 -> IO_ReadDigitalInput4/2, IO_ReadDigitalInput4/1
  Ground5/1 -> IO_ReadDigitalInput5/2, IO_ReadDigitalInput5/1
  Ground6/1 -> IO_ReadDigitalInput6/1, IO_ReadDigitalInput6/2
  Ground7/1 -> IO_ReadDigitalInput7/2, IO_ReadDigitalInput7/1
  Ground8/1 -> IO_ReadDigitalInput15/2, IO_ReadDigitalInput15/1
  Ground9/1 -> IO_ReadDigitalInput17/1, IO_ReadDigitalInput17/2
  Ground10/1 -> IO_ReadDigitalInput8/1, IO_ReadDigitalInput8/2
  Ground11/1 -> IO_ReadDigitalInput9/2, IO_ReadDigitalInput9/1
  IO_ReadDigitalInput2/2 -> Terminator2/1
  IO_ReadDigitalInput3/2 -> Terminator3/1
  IO_ReadDigitalInput4/2 -> Terminator4/1
  IO_ReadDigitalInput5/2 -> Terminator5/1
  IO_ReadDigitalInput6/2 -> Terminator6/1
  IO_ReadDigitalInput7/2 -> Terminator7/1
  IO_ReadDigitalInput15/2 -> Terminator8/1
  IO_ReadDigitalInput17/2 -> Terminator9/1
  IO_ReadDigitalInput8/2 -> Terminator10/1
  IO_ReadDigitalInput9/2 -> Terminator11/1
  IO_ReadDigitalInput10/2 -> Terminator12/1
  IO_ReadDigitalInput11/2 -> Terminator13/1
  IO_ReadDigitalInput12/2 -> Terminator14/1
  IO_ReadDigitalInput13/2 -> Terminator15/1
  IO_ReadDigitalInput14/2 -> Terminator16/1
  IO_ReadDigitalInput16/2 -> Terminator17/1
  IO_ReadDigitalInput18/2 -> Terminator18/1
  Ground12/1 -> IO_ReadDigitalInput10/1, IO_ReadDigitalInput10/2
  Ground13/1 -> IO_ReadDigitalInput11/2, IO_ReadDigitalInput11/1
  Ground14/1 -> IO_ReadDigitalInput12/1, IO_ReadDigitalInput12/2
  Ground15/1 -> IO_ReadDigitalInput13/1, IO_ReadDigitalInput13/2
  Ground16/1 -> IO_ReadDigitalInput14/1, IO_ReadDigitalInput14/2
  Ground17/1 -> IO_ReadDigitalInput16/2, IO_ReadDigitalInput16/1
  Ground18/1 -> IO_ReadDigitalInput18/1, IO_ReadDigitalInput18/2
  Gain20/1 -> Add2/4
  Gain18/1 -> Add2/6
  Gain19/1 -> Add2/5
  Gain25/1 -> Add2/13
  Gain29/1 -> Add2/9
  Gain30/1 -> Add2/8
  Gain31/1 -> Add2/7
  Gain21/1 -> Add2/3
  Gain17/1 -> Add2/15
  Data Type Conversion2/1 -> LSD_Data2/1
  Gain28/1 -> Add2/10
  Add2/1 -> Data Type Conversion2/1
  Gain16/1 -> Add2/16
  Gain26/1 -> Add2/12
  Gain27/1 -> Add2/11
  Gain22/1 -> Add2/2
  Gain23/1 -> Add2/1
  Constant1/1 -> Gain30/1, Gain22/1, Gain20/1, Gain18/1, Gain28/1, Gain16/1, Gain24/1, Gain26/1
  Gain24/1 -> Add2/14
  Ground19/1 -> IO_ReadPwm/1, IO_ReadPwm/2
  IO_ReadPwm/1 -> PWM_IN_P13_Freq/1
  IO_ReadPwm/2 -> PWM_IN_P13_Duty/1
  LSD8/1 -> Terminator19/1
  LSD7/1 -> Terminator20/1
  LSD6/1 -> Terminator21/1
  LSD1/1 -> Terminator27/1
  LSD2/1 -> Terminator26/1
  LSD3/1 -> Terminator25/1
  LSD5/1 -> Terminator22/1
  LSD4/1 -> Terminator24/1
  Constant2/1 -> Gain7/1, Gain1/1, Gain3/1, Gain5/1, Gain9/1, Gain11/1, Gain13/1, Gain15/1
  LSD12/1 -> Terminator31/1
  LSD16/1 -> Terminator23/1
  LSD11/1 -> Terminator32/1
  LSD13/1 -> Terminator30/1
  LSD14/1 -> Terminator29/1
  LSD15/1 -> Terminator28/1
  LSD10/1 -> Terminator33/1
  LSD9/1 -> Terminator34/1
  Constant3/1 -> Gain17/1, Gain25/1, Gain27/1, Gain29/1, Gain31/1, Gain19/1, Gain23/1, Gain21/1
  P90/1 -> Terminator35/1
  P91/1 -> Terminator36/1
  P22/1 -> Terminator38/1
  P24/1 -> Terminator40/1
  P34/1 -> Terminator42/1
  P33/1 -> Terminator41/1
  P21/1 -> Terminator39/1
  P20/1 -> Terminator37/1
  P15/1 -> Terminator44/1
  P16/1 -> Terminator43/1
  Constant4/1 -> IO_WriteDigitalOutput9/1, IO_WriteDigitalOutput8/1, IO_WriteDigitalOutput7/1, IO_WriteDigitalOutput6/1, IO_WriteDigitalOutput5/1, IO_WriteDigitalOutput4/1, IO_WriteDigitalOutput3/1, IO_WriteDigitalOutput/1, IO_WriteDigitalOutput1/1, IO_WriteDigitalOutput2/1
  P40/1 -> Terminator45/1
  P94/1 -> Terminator51/1
  P93/1 -> Terminator50/1
  P92/1 -> Terminator49/1
  P43/1 -> Terminator48/1
  P42/1 -> Terminator46/1
  Constant5/1 -> IO_WriteDigitalOutput15/1, IO_WriteDigitalOutput14/1, IO_WriteDigitalOutput13/1, IO_WriteDigitalOutput11/1, IO_WriteDigitalOutput10/1, IO_WriteDigitalOutput12/1
  Frequency/1 -> Terminator47/1
  Duty_Cycle/1 -> Terminator52/1
  IO_ReadPwm1/2 -> PWM_IN_P14_Duty/1
  IO_ReadPwm1/1 -> PWM_IN_P14_Freq/1
  Ground20/1 -> IO_ReadPwm1/2, IO_ReadPwm1/1
  Ground21/1 -> IO_ReadPwm2/1, IO_ReadPwm2/2
  IO_ReadPwm2/1 -> PWM_IN_P62_Freq/1
  IO_ReadPwm2/2 -> PWM_IN_P62_Duty/1
  OdoReading1/1 -> Subsystem1/2(OdoReading1)
  OdoReading2/1 -> Subsystem1/5(OdoReading2)
  OdoReading3/1 -> Subsystem1/7(OdoReading3)
  Subsystem1/9(ReadData) -> ReadData/1
  Subsystem1/8(Data_Count2) -> Data_Count2/1
  Eraseee/1 -> Subsystem1/4(Eraseee)
  Speed/1 -> Subsystem1/6(Speed)
  Subsystem1/14(D1) -> D1/1
  Subsystem1/15(D2) -> D2/1
  Subsystem1/16(D3) -> D3/1
  Subsystem1/3(Updated_Data) -> Updated_Data/1
  Subsystem1/11(A1) -> A1/1
  Subsystem1/12(A2) -> A2/1
  Subsystem1/13(A3) -> A3/1
  Subsystem1/1(RTE_Erase_Enable) -> RTE_Erase_Enable/1
  Subsystem1/2(Erase) -> Erase/1
  Subsystem1/4(RTE_Write_Enable) -> RTE_Write_Enable/1
  Subsystem1/5(Write) -> Write/1
  Subsystem1/7(DataCount) -> DataCount/1
  Ign/1 -> Subsystem1/3(Ign)
  Subsystem1/6(Readdata2) -> Readdata2/1
  Subsystem1/10(RTE_EEPROM_Value_Read) -> RTE_EEPROM_Value_Read/1
  RTE_EEPROM_Value_Write/1 -> Subsystem1/1(RTE_EEPROM_Value_Write)

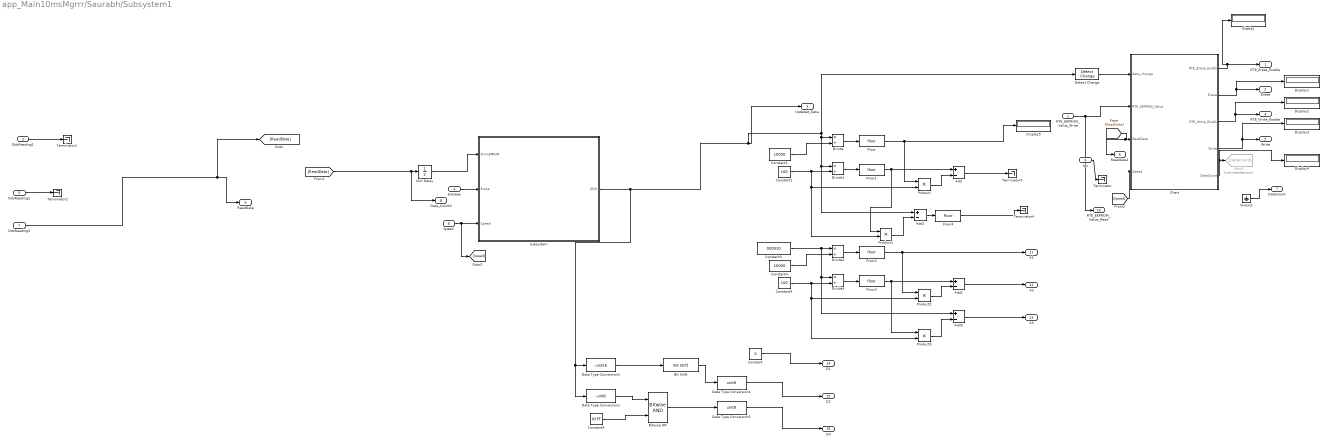
== system app_Main10msMgrrr/Saurabh/Subsystem1 ==
  RTE_EEPROM_Value_Write : Inport
  OdoReading1 : Inport  Port=2
  Ign : Inport  Port=3
  Eraseee : Inport  Port=4
  OdoReading2 : Inport  Port=5
  Speed : Inport  Port=6
  OdoReading3 : Inport  Port=7
  Add{,1..3} (4 alike) : Sum  Inputs=+-
  Bit Shift : hdlsllib/Logic and Bit Operations/Bit Shift  mode=Shift Right Logical  N=8
      settings: SourceProductName=Simulink
  Bitwise OR : simulink/Logic and Bit Operations/Bitwise Operator  logicop=AND  UseBitMask=off  NumInputPorts=2  BitMask=bin2dec('11011001')  BitMaskRealWorld=Stored Integer
  Chart : Stateflow chart  BlockKeywords=__PRM__SERIALIZED__DATA__:Stateflow Chart,Stateflow Diagram  TreatAsAtomicUnit=on
  Constant : Constant  Value=0
  Constant1 : Constant  Value=10000
  Constant2 : Constant  Value=100
  Constant3 : Constant  Value=000010
  Constant4 : Constant  Value=10000
  Constant5 : Constant  Value=100
  Constant6 : Constant  Value=0XFF  OutDataTypeStr=uint8
  Data Type Conversion1 : DataTypeConversion  OutDataTypeStr=uint8
  Data Type Conversion2 : DataTypeConversion  OutDataTypeStr=uint16
  Data Type Conversion4 : DataTypeConversion  OutDataTypeStr=uint8
  Data Type Conversion5 : DataTypeConversion  OutDataTypeStr=uint8
  Detect Change : simulink/Logic and Bit Operations/Detect Change  vinit=0  OutDataTypeStr=boolean
  Display{,1..5} (6 alike) : Display
  Divide{,1..3} (4 alike) : Product  Inputs=*/
  Floor{,1..4} (5 alike) : Rounding
  Goto1 : Goto  Commented=on  GotoTag=DataCount
  Ground : Ground
  Product{,1..3} (4 alike) : Product
  Subsystem : Subsystem
  Terminator{,1..4} (5 alike) : Terminator
  Unit Delay : UnitDelay  SampleTime=-1  HasFrameUpgradeWarning=on
  RTE_Erase_Enable : Outport
  Erase : Outport  Port=2
  Updated_Data : Outport  Port=3
  RTE_Write_Enable : Outport  Port=4
  Write : Outport  Port=5
  Readdata2 : Outport  Port=6
  DataCount : Outport  Port=7
  Data_Count2 : Outport  Port=8
  ReadData : Outport  Port=9
  RTE_EEPROM_Value_Read : Outport  Port=10
  A1 : Outport  Port=11
  A2 : Outport  Port=12
  A3 : Outport  Port=13
  D1 : Outport  Port=14
  D2 : Outport  Port=15
  D3 : Outport  Port=16
  wires:
  Floor1/1 -> Product1/1, Add/1
  Product3/1 -> Add3/2
  RTE_EEPROM_Value_Write/1 -> Chart/2(RTE_EEPROM_Value), RTE_EEPROM_Value_Read/1
  Divide/1 -> Floor/1
  Data Type Conversion1/1 -> Bitwise OR/1
  OdoReading2/1 -> Terminator2/1
  Constant5/1 -> Product2/2, Product3/2, Divide3/2
  Speed/1 -> [Speed], Subsystem/3(Speed)
  Bit Shift/1 -> Data Type Conversion4/1
  Constant6/1 -> Bitwise OR/2
  Data Type Conversion2/1 -> Bit Shift/1
  [ReadData] -> Readdata2/1, Chart/3(ReadData)
  Floor4/1 -> Terminator4/1
  Add/1 -> Terminator3/1
  Chart/5(DataCount) -> Display4/1, Goto1/1
  OdoReading1/1 -> Terminator1/1
  Data Type Conversion5/1 -> D3/1
  Constant/1 -> D1/1
  Data Type Conversion4/1 -> D2/1
  Divide3/1 -> Floor3/1
  Bitwise OR/1 -> Data Type Conversion5/1
  Ground/1 -> DataCount/1
  Ign/1 -> Terminator/1
  Subsystem/1(ODO) -> Data Type Conversion2/1, Data Type Conversion1/1, Updated_Data/1, Add1/1, Divide1/1, Divide/1, Detect Change/1
  Chart/3(RTE_Write_Enable) -> RTE_Write_Enable/1, Display2/1
  Constant2/1 -> Divide1/2, Product1/2, Product/2
  Constant4/1 -> Divide2/2
  [ReadData] -> Data_Count2/1, Unit Delay/1
  Floor/1 -> Display5/1, Product/1
  [Speed] -> Chart/4(Speed)
  OdoReading3/1 -> ReadData/1, [ReadData]
  Divide2/1 -> Floor2/1
  Eraseee/1 -> Subsystem/2(Erase)
  Constant1/1 -> Divide/2
  Detect Change/1 -> Chart/1(data_change)
  Chart/2(Erase) -> Erase/1, Display1/1
  Unit Delay/1 -> Subsystem/1(FromEPROM)
  Floor2/1 -> A1/1, Product2/1
  Chart/1(RTE_Erase_Enable) -> RTE_Erase_Enable/1, Display/1
  Product/1 -> Add/2
  Floor3/1 -> Add2/1, Product3/1
  Product2/1 -> Add2/2
  Product1/1 -> Add1/2
  Constant3/1 -> Divide2/1, Divide3/1, Add3/1
  Add2/1 -> A2/1
  Add1/1 -> Floor4/1
  Add3/1 -> A3/1
  Chart/4(Write) -> Write/1, Display3/1
  Divide1/1 -> Floor1/1

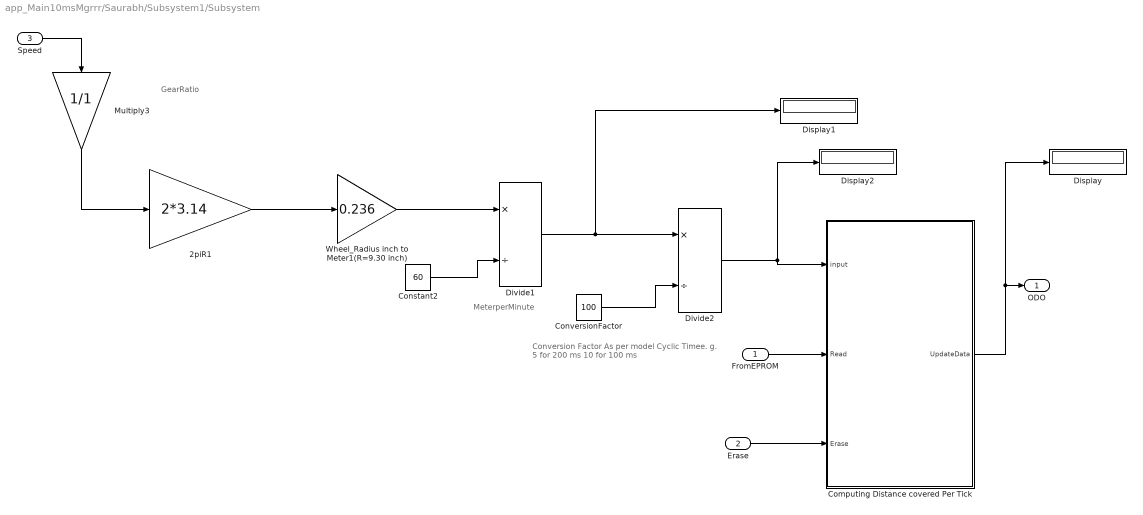
== system app_Main10msMgrrr/Saurabh/Subsystem1/Subsystem ==
  note: GearRatio
  note: Conversion Factor As per model Cyclic Timee.
      | g. 5 for 200 ms
      | 10 for 100 ms
  note: MeterperMinute
  FromEPROM : Inport
  Erase : Inport  Port=2
  Speed : Inport  Port=3
  2piR1 : Gain  Gain=2*3.14  OutDataTypeStr=int16  LockScale=on
  Computing Distance covered Per Tick : Stateflow chart  TreatAsAtomicUnit=on
  Constant2 : Constant  Value=60
  ConversionFactor : Constant  Value=100  OutDataTypeStr=double
  Display : Display
  Display1 : Display
  Display2 : Display
  Divide1 : Product  Inputs=*/
  Divide2 : Product  Inputs=*/
  Multiply3 : Gain  Gain=1/1
  Wheel_Radius inch to Meter1(R=9.30 inch) : Gain  Gain=0.236  OutDataTypeStr=int16  LockScale=on
  ODO : Outport
  wires:
  Divide1/1 -> Display1/1, Divide2/1
  ConversionFactor/1 -> Divide2/2
  Multiply3/1 -> 2piR1/1
  Wheel_Radius inch to Meter1(R=9.30 inch)/1 -> Divide1/1
  Constant2/1 -> Divide1/2
  2piR1/1 -> Wheel_Radius inch to Meter1(R=9.30 inch)/1
  Divide2/1 -> Display2/1, Computing Distance covered Per Tick/1(input)
  Computing Distance covered Per Tick/1(UpdateData) -> Display/1, ODO/1
  FromEPROM/1 -> Computing Distance covered Per Tick/2(Read)
  Erase/1 -> Computing Distance covered Per Tick/3(Erase)
  Speed/1 -> Multiply3/1

== stateflow chart app_Main10msMgrrr/Saurabh/Subsystem1/Chart ==
  state Read [commented out]
    state Read1 [commented out]
      en:
    state Read2 [commented out]
      en:
    state Read3 [commented out]
      en:
    (default) -> Read1 [commented out]
    Read1 -> Read2 [commented out]
    Read2 -> Read3 [commented out]
  state Init
    RTE_Erase_Enable = 0;
    Erase = 0;
    RTE_Write_Enable = 0;
    Write = 0;
  state ReadFormat
    en:
    DataCount=ReadData;
  state Write
    state Erase
      en:
      RTE_Erase_Enable = 1;
    state Erase1
      en:
      RTE_Erase_Enable = 0;
    state Erase2
      en:
      Erase = 1;
    state Erase3
      en:
      Erase = 0;
    state Write
      en:
      RTE_Write_Enable = 1;
    state Write1
      en:
      RTE_Write_Enable = 0;
    state Write2
      en:
      Write = 1;
    state Write3
      en:
      Write = 0;
    (default) -> Erase
    (junction 47) -> Erase
    (junction 45) -> (junction 47) : [data_change]
    Erase -> Erase1 : after(500, msec)
    Erase1 -> Erase2 : after(500, msec)
    Erase2 -> Erase3 : after(500, msec)
    Erase3 -> Write.Write : after(500, msec)
    Write.Write -> Write1 : after(500, msec)
    Write1 -> Write2 : after(500, msec)
    Write2 -> Write3 : after(500, msec)
    Write3 -> (junction 45) [order 2] : [after(500, msec)]
  state SameValue [commented out]
    en:
    RTE_Write_Enable = 0;
    RTE_Erase_Enable = 0;
  (default) -> Read [commented out]
  (default) -> Init
  Write3 -> Init [order 1] : [~Speed]
  Init -> (junction 76) : [after(500,msec)]
  (junction 76) -> ReadFormat : [Speed>0 && data_change ]
  ReadFormat -> Write : [after(500,msec)]
  Read3 -> (junction 16) [commented out]
  (junction 16) -> ? [commented out] : [RTE_EEPROM_Value ~= data_change]
  (junction 16) -> SameValue [commented out]
  data: RTE_Erase_Enable output; data_change input; RTE_EEPROM_Value input; Erase output =0; RTE_Write_Enable output =0; Write output =0; DataCount output =0; ReadData input; Speed input

== stateflow chart app_Main10msMgrrr/Saurabh/Subsystem1/Subsystem/Computing Distance covered Per Tick ==
  state Default
    state Default
      UpdateData=Read;
    state step1
      UpdateData=UpdateData+input;
    (default) -> Default.Default
    Default.Default -> step1 : [after(500,msec)]
    step1 -> step1
  state Erase
    UpdateData=20;
  (default) -> Default
  Erase -> Default : [~Erase]
  Default -> Erase : [Erase]
  data: input input; UpdateData output =0; Read input; Erase input
